simulink model "CHB"  (R2023a)
settings: Solver=VariableStepAuto  StartTime=0.0  StopTime=0.2  MaxStep=max_step_size  RelTol=1e-4  AbsTol=1e-5
undefined symbols (not defined in the file): plecs, Ts
libraries: plecslib x14
settings Model: Creator=lokit  LastModifiedBy=lokit

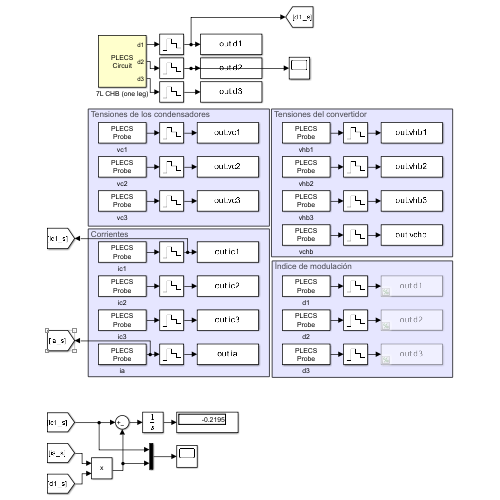
[thumbnail: Simulink's stored preview of the top-level diagram]
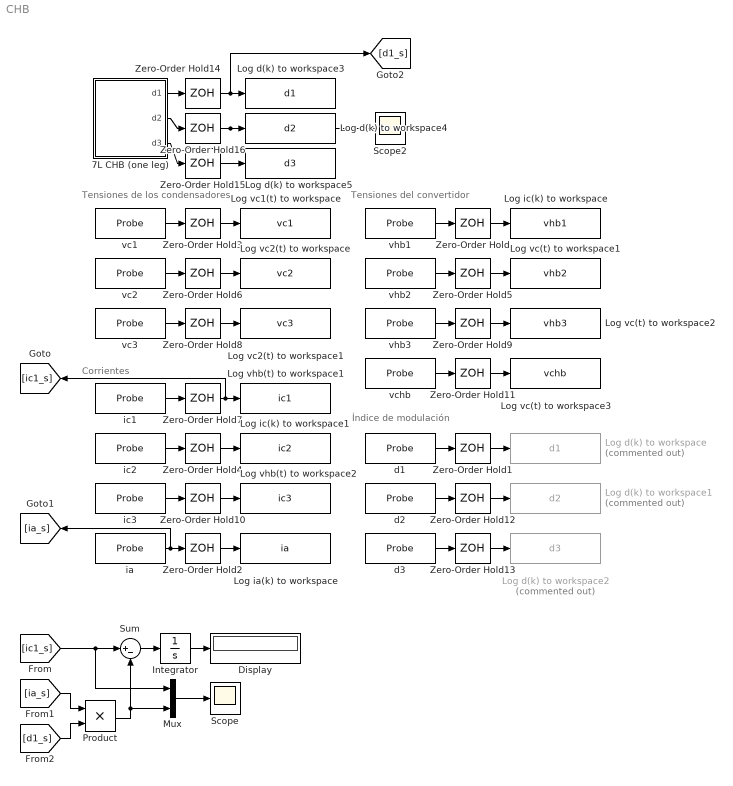
== system CHB ==
  note: Índice de modulación
  note: Tensiones de los condensadores
  note: Tensiones del convertidor
  note: Corrientes
  7L CHB (one leg) : Subsystem  LoadFcn=plecs('sl', 200);  InitFcn=plecs('sl', 214);  StartFcn=plecs('sl', 208);  StopFcn=plecs('sl', 209);  mask(PlecsCircuit){PLECSData=<binary blob, 12108 chars, not shown>}
      mask prompts: PLECSData "PLECS Data (Do not delete or modify!)"
      mask init:
      | % PLACE CUSTOM INITIALIZATIONS ABOVE
      | % DO NOT REMOVE
      | plecs('sl', 215);
      | % DO NOT REMOVE
      settings: CopyFcn=plecs('sl', 203);  DeleteFcn=plecs('sl', 205);  UndoDeleteFcn=plecs('sl', 206);  PreSaveFcn=plecs('sl', 211);  PostSaveFcn=plecs('sl', 201);  NameChangeFcn=plecs('sl', 210);  DestroyFcn=plecs('sl', 207);  PreCopyFcn=plecs('sl', 216);  OpenFcn=plecs('sl', 202);  ErrorFcn=plerrorfcn
      mask Help: eval('plecs(''help'', ''qthelp:///creatingacircuit.html'')')
      mask Display: disp('PLECS\nCircuit')
  Display : Display
  Integrator : Integrator
  Log d(k) to workspace : ToWorkspace  Commented=on  VariableName=d1  SaveFormat=Timeseries  SampleTime=-1
  Log d(k) to workspace1 : ToWorkspace  Commented=on  VariableName=d2  SaveFormat=Timeseries  SampleTime=-1
  Log d(k) to workspace2 : ToWorkspace  Commented=on  VariableName=d3  SaveFormat=Timeseries  SampleTime=-1
  Log d(k) to workspace3 : ToWorkspace  VariableName=d1  SaveFormat=Timeseries  SampleTime=-1
  Log d(k) to workspace4 : ToWorkspace  VariableName=d2  SaveFormat=Timeseries  SampleTime=-1
  Log d(k) to workspace5 : ToWorkspace  VariableName=d3  SaveFormat=Timeseries  SampleTime=-1
  Log ia(k) to workspace : ToWorkspace  VariableName=ia  SaveFormat=Timeseries  SampleTime=-1
  Log ic(k) to workspace : ToWorkspace  VariableName=vhb1  SaveFormat=Timeseries  SampleTime=-1
  Log ic(k) to workspace1 : ToWorkspace  VariableName=ic2  SaveFormat=Timeseries  SampleTime=-1
  Log vc(t) to workspace1 : ToWorkspace  VariableName=vhb2  SaveFormat=Timeseries  SampleTime=-1
  Log vc(t) to workspace2 : ToWorkspace  VariableName=vhb3  SaveFormat=Timeseries  SampleTime=-1
  Log vc(t) to workspace3 : ToWorkspace  VariableName=vchb  SaveFormat=Timeseries  SampleTime=-1
  Log vc1(t) to workspace : ToWorkspace  VariableName=vc1  SaveFormat=Timeseries  SampleTime=-1
  Log vc2(t) to workspace : ToWorkspace  VariableName=vc2  SaveFormat=Timeseries  SampleTime=-1
  Log vc2(t) to workspace1 : ToWorkspace  VariableName=vc3  SaveFormat=Timeseries  SampleTime=-1
  Log vhb(t) to workspace1 : ToWorkspace  VariableName=ic1  SaveFormat=Timeseries  SampleTime=-1
  Log vhb(t) to workspace2 : ToWorkspace  VariableName=ic3  SaveFormat=Timeseries  SampleTime=-1
  Mux : Mux  Inputs=2
  Product : Product
  Scope : Scope
  Scope2 : Scope
  Sum : Sum  Inputs=|+-
  Zero-Order Hold{,1..16} (17 alike) : ZeroOrderHold  SampleTime=Ts
  d1 : plecslib/Probe  tagno=3
      settings: SourceProductName=PLECS
  d2 : plecslib/Probe  tagno=15
      settings: SourceProductName=PLECS
  d3 : plecslib/Probe  tagno=16
      settings: SourceProductName=PLECS
  ia : plecslib/Probe  tagno=4
      settings: SourceProductName=PLECS
  ic1 : plecslib/Probe  tagno=8
      settings: SourceProductName=PLECS
  ic2 : plecslib/Probe  tagno=6
      settings: SourceProductName=PLECS
  ic3 : plecslib/Probe  tagno=11
      settings: SourceProductName=PLECS
  vc1 : plecslib/Probe  tagno=1
      settings: SourceProductName=PLECS
  vc2 : plecslib/Probe  tagno=5
      settings: SourceProductName=PLECS
  vc3 : plecslib/Probe  tagno=9
      settings: SourceProductName=PLECS
  vchb : plecslib/Probe  tagno=12
      settings: SourceProductName=PLECS
  vhb1 : plecslib/Probe  tagno=2
      settings: SourceProductName=PLECS
  vhb2 : plecslib/Probe  tagno=7
      settings: SourceProductName=PLECS
  vhb3 : plecslib/Probe  tagno=10
      settings: SourceProductName=PLECS
  wires:
  vhb1/1 -> Zero-Order Hold/1
  ia/1 -> [ia_s], Zero-Order Hold2/1
  vc2/1 -> Zero-Order Hold6/1
  vc1/1 -> Zero-Order Hold3/1
  Zero-Order Hold3/1 -> Log vc1(t) to workspace/1
  Zero-Order Hold/1 -> Log ic(k) to workspace/1
  d1/1 -> Zero-Order Hold1/1
  Zero-Order Hold4/1 -> Log ic(k) to workspace1/1
  Zero-Order Hold5/1 -> Log vc(t) to workspace1/1
  vhb2/1 -> Zero-Order Hold5/1
  ic2/1 -> Zero-Order Hold4/1
  Zero-Order Hold6/1 -> Log vc2(t) to workspace/1
  Zero-Order Hold9/1 -> Log vc(t) to workspace2/1
  vhb3/1 -> Zero-Order Hold9/1
  vc3/1 -> Zero-Order Hold8/1
  Zero-Order Hold8/1 -> Log vc2(t) to workspace1/1
  ic3/1 -> Zero-Order Hold10/1
  Zero-Order Hold10/1 -> Log vhb(t) to workspace2/1
  vchb/1 -> Zero-Order Hold11/1
  Zero-Order Hold11/1 -> Log vc(t) to workspace3/1
  d2/1 -> Zero-Order Hold12/1
  d3/1 -> Zero-Order Hold13/1
  Zero-Order Hold1/1 -> Log d(k) to workspace/1
  Zero-Order Hold12/1 -> Log d(k) to workspace1/1
  ic1/1 -> Zero-Order Hold7/1
  Zero-Order Hold13/1 -> Log d(k) to workspace2/1
  7L CHB (one leg)/1(d1) -> Zero-Order Hold14/1
  7L CHB (one leg)/2(d2) -> Zero-Order Hold16/1
  7L CHB (one leg)/3(d3) -> Zero-Order Hold15/1
  Zero-Order Hold15/1 -> Log d(k) to workspace5/1
  Zero-Order Hold16/1 -> Scope2/1, Log d(k) to workspace4/1
  Zero-Order Hold2/1 -> Log ia(k) to workspace/1
  Zero-Order Hold14/1 -> [d1_s], Log d(k) to workspace3/1
  Zero-Order Hold7/1 -> [ic1_s], Log vhb(t) to workspace1/1
  [ia_s] -> Product/1
  [d1_s] -> Product/2
  Product/1 -> Mux/2, Sum/2
  [ic1_s] -> Mux/1, Sum/1
  Sum/1 -> Integrator/1
  Integrator/1 -> Display/1
  Mux/1 -> Scope/1

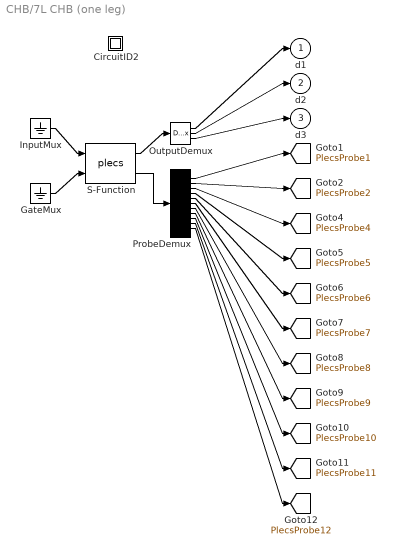
== system CHB/7L CHB (one leg) ==
  " CircuitID2 " : Subsystem
  " GateMux " : Ground
  " InputMux " : Ground
  " OutputDemux " : Demux  Outputs=[ 1 1 1 ]
  " ProbeDemux " : Demux  Outputs=[ 1 1 1 1 1 1 1 1 1 1 1 ]
  " S-Function " : S-Function  FunctionName=plecs  SFunctionDeploymentMode=off  EnableBusSupport=off
  d1 : Outport  PortDimensions=1
  d2 : Outport  Port=2  PortDimensions=1
  d3 : Outport  Port=3  PortDimensions=1
  tag scope: PlecsProbe10=global, PlecsProbe11=global, PlecsProbe12=global, PlecsProbe1=global, PlecsProbe2=global, PlecsProbe4=global, PlecsProbe5=global, PlecsProbe6=global, PlecsProbe7=global, PlecsProbe8=global, PlecsProbe9=global
  wires:
  " InputMux "/1 -> " S-Function "/1
  " GateMux "/1 -> " S-Function "/2
  " S-Function "/1 -> " OutputDemux "/1
  " S-Function "/2 -> " ProbeDemux "/1
  " OutputDemux "/1 -> d1/1
  " OutputDemux "/2 -> d2/1
  " OutputDemux "/3 -> d3/1
  " ProbeDemux "/1 -> [PlecsProbe1]
  " ProbeDemux "/2 -> [PlecsProbe2]
  " ProbeDemux "/3 -> [PlecsProbe4]
  " ProbeDemux "/4 -> [PlecsProbe5]
  " ProbeDemux "/5 -> [PlecsProbe6]
  " ProbeDemux "/6 -> [PlecsProbe7]
  " ProbeDemux "/7 -> [PlecsProbe8]
  " ProbeDemux "/8 -> [PlecsProbe9]
  " ProbeDemux "/9 -> [PlecsProbe10]
  " ProbeDemux "/10 -> [PlecsProbe11]
  " ProbeDemux "/11 -> [PlecsProbe12]

== system CHB/7L CHB (one leg)/ CircuitID2  ==
